simulink model "impulse_ex_2c"  (R2024a)
settings: Solver=VariableStepAuto  StartTime=0.0  StopTime=6.23456  RelTol=1e-6  AbsTol=1e-6
values from neighbouring files (symbols this model uses):
  dt = 0.01    [impulseDD.sldd]
undefined symbols (not defined in the file or in its folder): Call, Function, sys
libraries: simulink x1
settings Model: DataDictionary=impulseDD.sldd  Creator=grouleau  LastModifiedBy=grouleau

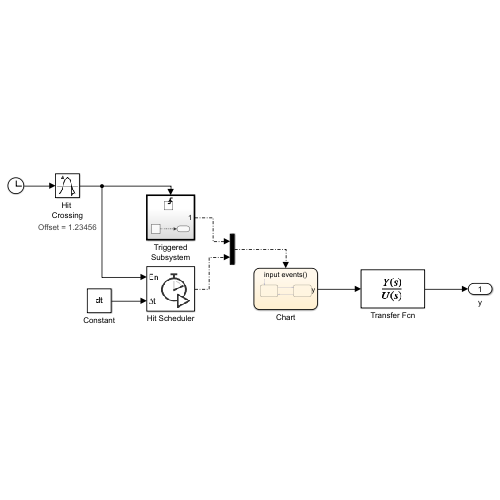
[thumbnail: Simulink's stored preview of the top-level diagram]
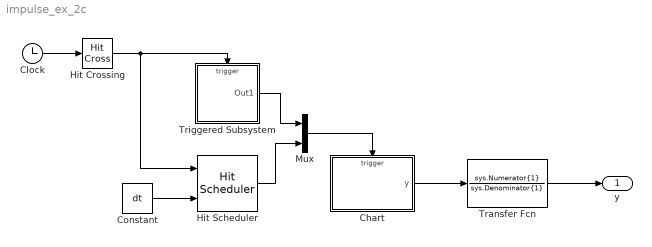
== system impulse_ex_2c ==
  Chart : Stateflow chart  TreatAsAtomicUnit=on
  Clock : Clock
  Constant : Constant  Value=dt
  Hit Crossing : HitCross  HitCrossingOffset=1.23456
      settings: AttributesFormatString=Offset = %<HitCrossingOffset>
  Hit Scheduler : HitScheduler  HitSchedulerOutputType=Function-Call
  Mux : Mux  Inputs=2
  Transfer Fcn : TransferFcn  Numerator=sys.Numerator{1}  Denominator=sys.Denominator{1}
  Triggered Subsystem : Subsystem  TreatAsAtomicUnit=on
  y : Outport
  wires:
  Chart/1(y) -> Transfer Fcn/1
  Transfer Fcn/1 -> y/1
  Clock/1 -> Hit Crossing/1
  Constant/1 -> Hit Scheduler/2
  Hit Crossing/1 -> Hit Scheduler/1, Triggered Subsystem/Trigger
  Triggered Subsystem/1(Out1) -> Mux/1
  Hit Scheduler/1 -> Mux/2
  Mux/1 -> Chart/Trigger

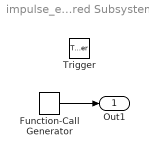
== system impulse_ex_2c/Triggered Subsystem ==
  Trigger : TriggerPort  VariantControl=(inherit)
  Function-Call Generator : simulink/Ports & Subsystems/Function-Call Generator  sample_time=-1  numberOfIterations=1  DisallowWideOutput=off
  Out1 : Outport
  wires:
  Function-Call Generator/1 -> Out1/1

== stateflow chart impulse_ex_2c/Chart ==
  settings: executeAtInitialization=1
  state off
    en:y=0;
  state on
    en: y=1/dt;
  (default) -> off
  off -> on : TrigOn
  on -> off : TrigOff
  data: y output; dt parameter
  events: TrigOn input FUNCTION_CALL_EVENT; TrigOff input FUNCTION_CALL_EVENT
